simulink model "RIN251230_16_SV_H4_l2_2"  (R2018b)
settings: Solver=VariableStepAuto  StartTime=0.0  StopTime=0.2  RelTol=1e-3
libraries: powerlib x83, powerlib_meascontrol x4
settings Model: Creator=ADMINISTRATOR  LastModifiedBy=VID Company
settings SFSimCC: SimUseLocalCustomCode=off
settings RTWCC: RTWUseLocalCustomCode=off
settings CodeAppCC: StateflowObjectComments=on
settings SimscapeCC: SimscapeNormalizeSystem=off

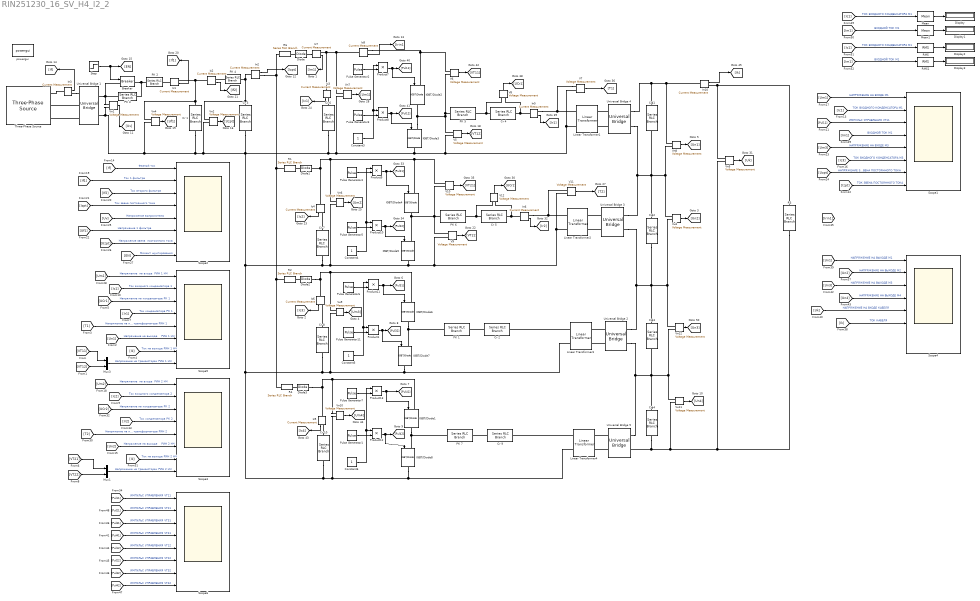
== system RIN251230_16_SV_H4_l2_2 ==
   R{1..2,4,6} (4 alike) : powerlib/Elements/Series RLC Branch  LConnTagsString=__new0  RConnTagsString=__new0  BranchType=R  Resistance=0.001  Inductance=1e-3  SetiL0=off  InitialCurrent=0  Capacitance=1e-6  Setx0=off  InitialVoltage=0  Measurements=None
      settings: SourceProductName=Simscape Electrical
  " R3" : powerlib/Elements/Series RLC Branch  LConnTagsString=__new0  RConnTagsString=__new0  BranchType=R  Resistance=100  Inductance=1e-3  SetiL0=off  InitialCurrent=0  Capacitance=1e-6  Setx0=off  InitialVoltage=0  Measurements=None
      settings: SourceProductName=Simscape Electrical
  Breaker : powerlib/Elements/Breaker  InitialState=0  SwitchingTimes="[1/60  5/60]"  External=on  BreakerResistance=0.0001  SnubberResistance=1e6  SnubberCapacitance=inf  Measurements=None  MoreParameters=on  NoBreakLoop=off
      settings: SourceProductName=Simscape Electrical
  Constant{3..6} (4 alike) : Constant
  Cr 1 : powerlib/Elements/Series RLC Branch  LConnTagsString=__new0  RConnTagsString=__new0  BranchType=C  Resistance=0.001  Inductance=5e-6  SetiL0=off  InitialCurrent=0  Capacitance=4100e-6  Setx0=off  InitialVoltage=0  Measurements=Branch voltage and current
      settings: SourceProductName=Simscape Electrical
  Cr {6..8,10} (4 alike) : powerlib/Elements/Series RLC Branch  LConnTagsString=__new0  RConnTagsString=__new0  BranchType=C  Resistance=0.001  Inductance=5e-6  SetiL0=off  InitialCurrent=0  Capacitance=120e-6  Setx0=off  InitialVoltage=0  Measurements=Branch voltage and current
      settings: SourceProductName=Simscape Electrical
  Cr {2,4..5,9} (4 alike) : powerlib/Elements/Series RLC Branch  LConnTagsString=__new0  RConnTagsString=__new0  BranchType=C  Resistance=0.001  Inductance=5e-6  SetiL0=off  InitialCurrent=0  Capacitance=1.6e-6  Setx0=off  InitialVoltage=0  Measurements=Branch voltage and current
      settings: SourceProductName=Simscape Electrical
  Cr 3 : powerlib/Elements/Series RLC Branch  LConnTagsString=__new0  RConnTagsString=__new0  BranchType=C  Resistance=0.001  Inductance=5e-6  SetiL0=off  InitialCurrent=0  Capacitance=10e-6  Setx0=off  InitialVoltage=0  Measurements=Branch voltage and current
      settings: SourceProductName=Simscape Electrical
  Diode{,1..3} (4 alike) : powerlib/Power Electronics/Diode  Ron=0.001  Lon=0  Vf=0.8  IC=0  UseSnubber=0  Rs=inf  Cs=250e-9  Measurements=off
  Display{,1..3} (4 alike) : Display
  IGBT/Diode{1..8} (8 alike) : powerlib/Power Electronics/IGBT//Diode  Ron=4.5e-6  Rs=1e5  Cs=inf  Measurements=off
      settings: SourceProductName=Simscape Electrical
  Ic{1..8} (8 alike) : powerlib/Measurements/Current Measurement  PhasorSimulation=off  OutputType=Complex  PSBequivalent=0
      settings: SourceProductName=Simscape Electrical
  Iн{2..3,5..6,10} (5 alike) : powerlib/Measurements/Current Measurement  PhasorSimulation=off  OutputType=Complex  PSBequivalent=0
      settings: SourceProductName=Simscape Electrical
  Linear Transformer{1..4} (4 alike) : powerlib/Elements/Linear Transformer  UNITS=pu  NominalPower=[ 20e3 16e3 ]  winding1=[250 1e-4 1e-7]  winding2=[500 1e-4 1e-7]  ThreeWindings=off  winding3=[3.15e+05 0.7938 0.084225]  RmLm=[1e4 1e4]  Measurements=None  DataType=off
      settings: SourceProductName=Simscape Electrical
  Mean : powerlib_meascontrol/Measurements/Mean  Freq=16000  Vinit=0  Ts=0
  Mean1 : powerlib_meascontrol/Measurements/Mean  Freq=16000  Vinit=0  Ts=0
  Mux1 : Mux  Inputs=2
  Mux3 : Mux  Inputs=2
  Product{1,7..13} (8 alike) : Product
  Pulse Generator1 : DiscretePulseGenerator  PulseType=Time based  Amplitude=20  Period=1/16e3  PulseWidth=27  PhaseDelay=1/64e3
  Pulse Generator11 : DiscretePulseGenerator  PulseType=Time based  Amplitude=20  Period=1/16e3  PulseWidth=27  PhaseDelay=3/64e3
  Pulse Generator2 : DiscretePulseGenerator  PulseType=Time based  Amplitude=20  Period=1/16e3  PulseWidth=27
  Pulse Generator3 : DiscretePulseGenerator  PulseType=Time based  Amplitude=20  Period=1/16e3  PulseWidth=27  PhaseDelay=1/32e3
  Pulse Generator4 : DiscretePulseGenerator  PulseType=Time based  Amplitude=20  Period=1/16e3  PulseWidth=27  PhaseDelay=1/32e3
  Pulse Generator5 : DiscretePulseGenerator  PulseType=Time based  Amplitude=20  Period=1/16e3  PulseWidth=27
  Pulse Generator6 : DiscretePulseGenerator  PulseType=Time based  Amplitude=20  Period=1/16e3  PulseWidth=27  PhaseDelay=1/64e3
  Pulse Generator7 : DiscretePulseGenerator  PulseType=Time based  Amplitude=20  Period=1/16e3  PulseWidth=27  PhaseDelay=3/64e3
  RMS : powerlib_meascontrol/Measurements/RMS  TrueRMS=on  Freq=16000  RMSInit=0  Ts=0
  RMS1 : powerlib_meascontrol/Measurements/RMS  TrueRMS=on  Freq=16000  RMSInit=0  Ts=0
  Scope{1..6} (6 alike) : Scope  NumInputPorts=8
  Step : Step  Time=0.03  SampleTime=0
  Three-Phase Source : powerlib/Electrical Sources/Three-Phase Source  InternalConnection=Yg  VoltagePhases=off  Voltage=380  PhaseAngle=0  Voltage_phases=[25e3 25e3 25e3]/sqrt(3)  PhaseAngles_phases=[0 -120 +120]  Frequency=50  NonIdealSource=on  SpecifyImpedance=off  Resistance=50e-3  Inductance=0.4e-3  ShortCircuitLevel=100e6  BaseVoltage=380  XRratio=7  BusType=swing  Pref=10e3  Qref=0  Prefabc=[10e3, 10e3, 10e3]  Qrefabc=[0, 0, 0]  Qmin=-inf  Qmax=inf
      settings: SourceProductName=Simscape Electrical
  Universal Bridge 1 : powerlib/Power Electronics/Universal Bridge  Arms=3  SnubberResistance=1000000  SnubberCapacitance=1e-12  Device=Diodes  Ron=1e-6  Lon=0  ForwardVoltages="[  0  0  ]"  ForwardVoltage=0  GTOparameters=[ 10e-6 , 20e-6 ]  IGBTparameters=[ 1e-6 , 2e-6 ]  Measurements=Device voltages  Measurements_2=None  converterType=Rectifier
      settings: SourceProductName=Simscape Electrical
  Universal Bridge {2..5} (4 alike) : powerlib/Power Electronics/Universal Bridge  Arms=2  SnubberResistance=1000000  SnubberCapacitance=1e-12  Device=Diodes  Ron=1e-6  Lon=0  ForwardVoltages="[  0  0  ]"  ForwardVoltage=0  GTOparameters=[ 10e-6 , 20e-6 ]  IGBTparameters=[ 1e-6 , 2e-6 ]  Measurements=None  Measurements_2=None  converterType=Rectifier
      settings: SourceProductName=Simscape Electrical
  V{5..12} (8 alike) : powerlib/Measurements/Voltage Measurement  PhasorSimulation=off  OutputType=Complex  PSBequivalent=0
      settings: SourceProductName=Simscape Electrical
  Vн{1..12} (12 alike) : powerlib/Measurements/Voltage Measurement  PhasorSimulation=off  OutputType=Complex  PSBequivalent=0
      settings: SourceProductName=Simscape Electrical
  powergui : powerlib/powergui  Priority=1  SimulationMode=Discrete  SampleTime=1e-7  frequency=60  Iterations=50  frequencyindice=0  Pbase=100e6  ErrMax=1e-4  UnitsV=kV  UnitsW=MW  buscounter=0  FunctionMessages=off  echomessages=off  EnableUseOfTLC=off  CurrentSourceSwitches=off  DisableSnubberDevices=off  DisableRonSwitches=off  DisableVfSwitches=off  DisplayEquations=off  SolverType=Tustin/Backward Euler (TBE)  Interpol=off  ExternalGateDelay=off  methode=off  Ts=100  x0status=blocks  SPID=off  SwTol=0  HookPort=off  RestoreLinks=warning  ResistiveCurrentMeasurement=off  Frange=[0:2:500]  Ylog=off  Xlog=on  ShowGrid=off  save=off  variable=ZData  structure=0  ZoomFFT=off  StartTime=0.0  cycles=1  DisplayStyle=1  fundamental=60  FreqAxis=off  MaxFrequency=1000  frequencyindicesteady=1  RmsSteady=1  display=off
  РК {1,5..7} (4 alike) : powerlib/Elements/Series RLC Branch  LConnTagsString=__new0  RConnTagsString=__new0  BranchType=RL  Resistance=0.000001  Inductance=13.6e-6  SetiL0=off  InitialCurrent=0  Capacitance=3e-6  Setx0=off  InitialVoltage=0  Measurements=None
      settings: SourceProductName=Simscape Electrical
  РК 2 : powerlib/Elements/Series RLC Branch  LConnTagsString=__new0  RConnTagsString=__new0  BranchType=RL  Resistance=1e-3  Inductance=1e-3  SetiL0=off  InitialCurrent=0  Capacitance=3e-6  Setx0=off  InitialVoltage=0  Measurements=None
      settings: SourceProductName=Simscape Electrical
  РК 3 : powerlib/Elements/Series RLC Branch  LConnTagsString=__new0  RConnTagsString=__new0  BranchType=RL  Resistance=2  Inductance=1e-6  SetiL0=off  InitialCurrent=0  Capacitance=3e-6  Setx0=off  InitialVoltage=0  Measurements=None
      settings: SourceProductName=Simscape Electrical
  РК 4 : powerlib/Elements/Series RLC Branch  LConnTagsString=__new0  RConnTagsString=__new0  BranchType=RL  Resistance=1e-3  Inductance=10e-6  SetiL0=off  InitialCurrent=0  Capacitance=3e-6  Setx0=off  InitialVoltage=0  Measurements=None
      settings: SourceProductName=Simscape Electrical
  Сф{1..4} (4 alike) : powerlib/Elements/Series RLC Branch  LConnTagsString=__new0  RConnTagsString=__new0  BranchType=C  Resistance=0.001  Inductance=5e-6  SetiL0=off  InitialCurrent=0  Capacitance=60e-6  Setx0=off  InitialVoltage=300  Measurements=Branch voltage and current
      settings: SourceProductName=Simscape Electrical
  wires:
  [UCr1] -> Scope5/3  "Напряжение на конденсаторе РК 1"
  [Ik] -> Scope5/7  "Ток на выходе РИН 1 НЧ"
  [Un1] -> Scope5/6  "Напряжение на выходе    РИН 1 НЧ"
  [T1] -> Scope5/5  "Напряжение на первичной обмотке трансформатора РИН 1"
  [Ir1] -> Scope5/4  "Ток конденсатора РК 1"
  Iн2/1 -> [Izpt]
  [Ic1] -> Scope5/2  "Ток входного конденсатора 1"
  Iн3/1 -> [If]
  Step/1 -> [EN], Breaker/1
  Vн2/1 -> [Uzpt]
  Vн4/1 -> [Uf1]
  Vн1/1 -> [Uv]
  Ic1/1 -> [If1]
  Ic2/1 -> [If2]
  [If] -> Scope2/1  "Фазный ток"
  [If1] -> Scope2/2  "Ток 1 фильтра"
  [If2] -> Scope2/3  "Ток второго фильтра"
  [Izpt] -> Scope2/4  "Ток звена постоянного тока"
  [Uv] -> Scope2/5  "Напряжение выпрямителя"
  [Uf1] -> Scope2/6  "Напряжение 1 фильтра"
  [Uzpt] -> Scope2/7  "Напряжение звена  постоянного тока"
  [EN] -> Scope2/8  "Момент шунтирования"
  [Um1] -> Scope5/1  "Напряжение  на входе  РИН 1 НЧ"
  [VT12] -> Mux3/2
  [VT11] -> Mux3/1
  Mux3/1 -> Scope5/8  "Напряжение на транзисторах РИН 1 НЧ"
  V6/1 -> [VT11]
  V5/1 -> [VT12]
  Vн5/1 -> [Uk]
  V7/1 -> [T1]
  V8/1 -> [UCr1]
  Iн5/1 -> [Ir1]
  Product8/1 -> IGBT/Diode3/1, [Pul12]
  Product7/1 -> IGBT/Diode2/1, [Pul11]
  Ic3/1 -> [Ic1]
  Pulse Generator2/1 -> Product7/2
  Pulse Generator3/1 -> Product8/2
  Constant3/1 -> Product7/1, Product8/1
  Vн7/1 -> [Um1]
  V10/1 -> [VT21]
  V9/1 -> [VT22]
  V11/1 -> [T2]
  V12/1 -> [UCr2]
  Iн6/1 -> [Ir2]
  Product10/1 -> IGBT/Diode5/1, [Pul22]
  Product9/1 -> IGBT/Diode4/1, [Pul21]
  Ic4/1 -> [Ic2]
  Pulse Generator4/1 -> Product9/2
  Pulse Generator5/1 -> Product10/2
  Constant4/1 -> Product9/1, Product10/1
  Vн6/1 -> [Um2]
  Vн8/1 -> [Un1]
  Vн3/1 -> [Un2]
  Iн10/1 -> [Ik]
  [UCr2] -> Scope3/3  "Напряжение на конденсаторе РК 2"
  [Ik] -> Scope3/7  "Ток на выходе РИН 2 НЧ"
  [Un2] -> Scope3/6  "Напряжение на выходе    РИН 2 НЧ"
  [T2] -> Scope3/5  "Напряжение на первичной обмотке трансформатора РИН 2"
  [Ir2] -> Scope3/4  "Ток конденсатора РК 2"
  [Ic2] -> Scope3/2  "Ток входного конденсатора 2"
  [Um2] -> Scope3/1  "Напряжение  на входе  РИН 2 НЧ"
  [VT22] -> Mux1/2
  [VT21] -> Mux1/1
  Mux1/1 -> Scope3/8  "Напряжение на транзисторах РИН 2 НЧ"
  Product1/1 -> [Pul32], IGBT/Diode7/1
  Product11/1 -> IGBT/Diode6/1, [Pul31]
  Ic6/1 -> [Ic3]
  Pulse Generator6/1 -> Product11/2
  Pulse Generator11/1 -> Product1/2
  Constant5/1 -> Product11/1, Product1/1
  Vн9/1 -> [Um3]
  Product12/1 -> [Pul42], IGBT/Diode8/1
  Product13/1 -> [Pul41], IGBT/Diode1/1
  Ic5/1 -> [Ic4]
  Pulse Generator7/1 -> Product13/2
  Pulse Generator1/1 -> Product12/2
  Constant6/1 -> Product13/1, Product12/1
  Vн10/1 -> [Um4]
  Vн12/1 -> [Un3]
  Vн11/1 -> [Un4]
  [Pul11] -> Scope1/3  "ИМПУЛЬС УПРАВЛЕНИЯ VT11"
  [Uzpt] -> Scope1/7  "НАПРЯЖЕНИЕ ЗВЕНА ПОСТОЯННОГО ТОКА"
  [Ic3] -> Scope1/6  "ТОК ВХОДНОГО КОНДЕНСАТОРА М3"
  [Um3] -> Scope1/5  "НАПРЯЖЕНИЕ НА ВХОДЕ М3"
  [Im1] -> Scope1/4  "ВХОДНОЙ ТОК М1"
  [Ic1] -> Scope1/2  "ТОК ВХОДНОГО КОНДЕНСАТОРА М1"
  [Um1] -> Scope1/1  "НАПРЯЖЕНИЕ НА ВХОДЕ М1"
  [Un3] -> Scope4/3  "НАПРЯЖЕНИЕ НА ВЫХОДЕ М3"
  [Ik] -> Scope4/6  "ТОК КАБЕЛЯ"
  [Uk] -> Scope4/5  "НАПРЯЖЕНИЕ НА ВХОДЕ КАБЕЛЯ"
  [Un4] -> Scope4/4  "НАПРЯЖЕНИЕ НА ВЫХОДЕ М4"
  [Un2] -> Scope4/2  "НАПРЯЖЕНИЕ НА ВЫХОДЕ М2"
  [Un1] -> Scope4/1  "НАПРЯЖЕНИЕ НА ВЫХОДЕ М1"
  [Izpt] -> Scope1/8  "ТОК ЗВЕНА ПОСТОЯННОГО ТОКА"
  Ic7/1 -> [Im1]
  [Pul11] -> Scope6/1  "ИМПУЛЬС УПРАВЛЕНИЯ VT11"
  [Pul21] -> Scope6/2  "ИМПУЛЬС УПРАВЛЕНИЯ VT21"
  [Pul41] -> Scope6/4  "ИМПУЛЬС УПРАВЛЕНИЯ VT41"
  [Pul31] -> Scope6/3  "ИМПУЛЬС УПРАВЛЕНИЯ VT31"
  [Pul12] -> Scope6/5  "ИМПУЛЬС УПРАВЛЕНИЯ VT12"
  [Pul22] -> Scope6/6  "ИМПУЛЬС УПРАВЛЕНИЯ VT22"
  [Pul32] -> Scope6/7  "ИМПУЛЬС УПРАВЛЕНИЯ VT32"
  [Pul42] -> Scope6/8  "ИМПУЛЬС УПРАВЛЕНИЯ VT42"
  Ic8/1 -> [Irin1]
  [Ic1] -> Mean/1  "ТОК ВХОДНОГО КОНДЕНСАТОРА М1"
  [Im1] -> Mean1/1  "ВХОДНОЙ ТОК М1"
  Mean/1 -> Display/1
  Mean1/1 -> Display1/1
  RMS/1 -> Display2/1
  RMS1/1 -> Display3/1
  [Ic1] -> RMS/1  "ТОК ВХОДНОГО КОНДЕНСАТОРА М1"
  [Im1] -> RMS1/1  "ВХОДНОЙ ТОК М1"
  connections:
  РК 2/LConn1 -- Breaker/RConn1 -- РК 3/RConn1
  Universal Bridge 1/LConn3 -- Three-Phase Source/RConn3
  Universal Bridge 1/LConn2 -- Three-Phase Source/RConn2
  Iн3/LConn1 -- Three-Phase Source/RConn1
  Iн3/RConn1 -- Universal Bridge 1/LConn1
  Universal Bridge 1/RConn1 -- Vн1/LConn1 -- РК 3/LConn1 -- Breaker/LConn1
  Cr 1/LConn1 -- Vн4/LConn1 -- Ic2/LConn1 -- Ic1/RConn1
  Ic1/LConn1 -- РК 2/RConn1
  РК 4/LConn1 -- Ic2/RConn1
  IGBT/Diode3/LConn1 -- V6/LConn2 -- РК 5/LConn1 -- V5/LConn1 -- IGBT/Diode2/RConn1
  Iн5/LConn1 -- Cr 4/RConn1 -- V8/LConn2
  РК 5/RConn1 -- V8/LConn1 -- Cr 4/LConn1
  V7/LConn1 -- Iн5/RConn1 -- Linear Transformer1/LConn1
  IGBT/Diode3/RConn1 -- Linear Transformer1/LConn2 -- V7/LConn2 -- V5/LConn2 -- Linear Transformer3/LConn2 -- IGBT/Diode7/RConn1 -- Vн9/LConn2 -- Cr 8/RConn1 -- Cr 10/RConn1 -- Linear Transformer4/LConn2 -- IGBT/Diode8/RConn1 -- Vн10/LConn2 -- V11/LConn2 -- Linear Transformer2/LConn2 -- V9/LConn2 -- IGBT/Diode5/RConn1 -- Vн6/LConn2 -- Cr 7/RConn1 -- Cr 1/RConn1 -- Vн1/LConn2 -- Universal Bridge 1/RConn2 -- Vн4/LConn2 -- Vн2/LConn2 -- Cr 3/RConn1 -- Cr 6/RConn1 -- Vн7/LConn2
  V6/LConn1 -- IGBT/Diode2/LConn1 -- Ic8/RConn1
  V12/LConn2 -- Iн6/LConn1 -- Cr 5/RConn1
  Cr 5/LConn1 -- РК 6/RConn1 -- V12/LConn1
  Linear Transformer2/LConn1 -- V11/LConn1 -- Iн6/RConn1
  Сф2/RConn1 -- Сф3/LConn1 -- Universal Bridge 2/RConn1 -- Universal Bridge 3/RConn2 -- Vн12/LConn1 -- Vн3/LConn2
  Ic4/LConn1 -- Diode1/RConn1 -- Vн6/LConn1 -- V10/LConn1 -- IGBT/Diode4/LConn1
  Universal Bridge 3/RConn1 -- Universal Bridge 4/RConn2 -- Vн3/LConn1 -- Vн8/LConn2 -- Сф2/LConn1 -- Сф1/RConn1
  Universal Bridge 4/LConn2 -- Linear Transformer1/RConn2
  Cr 7/LConn1 -- Ic4/RConn1
  Universal Bridge 4/LConn1 -- Linear Transformer1/RConn1
  Cr 6/LConn1 -- Ic3/RConn1
  Universal Bridge 3/LConn1 -- Linear Transformer2/RConn1
  Universal Bridge 3/LConn2 -- Linear Transformer2/RConn2
  IGBT/Diode4/RConn1 -- IGBT/Diode5/LConn1 -- V9/LConn1 -- РК 6/LConn1 -- V10/LConn2
  Universal Bridge 4/RConn1 -- Iн10/LConn1 -- Vн8/LConn1 -- Сф1/LConn1
  Vн5/LConn1 -- " R3"/LConn1 -- Iн10/RConn1
  Cr 2/LConn1 -- РК 1/RConn1
  Vн9/LConn1 -- Diode2/RConn1 -- Ic6/LConn1 -- IGBT/Diode6/LConn1
  IGBT/Diode6/RConn1 -- IGBT/Diode7/LConn1 -- РК 1/LConn1
  Cr 8/LConn1 -- Ic6/RConn1
  Universal Bridge 2/LConn1 -- Linear Transformer3/RConn1
  Universal Bridge 2/LConn2 -- Linear Transformer3/RConn2
  Cr 9/LConn1 -- РК 7/RConn1
  Ic5/LConn1 -- Diode3/RConn1 -- Vн10/LConn1 -- IGBT/Diode1/LConn1
  РК 7/LConn1 -- IGBT/Diode8/LConn1 -- IGBT/Diode1/RConn1
  Universal Bridge 5/LConn1 -- Linear Transformer4/RConn1
  Universal Bridge 5/LConn2 -- Linear Transformer4/RConn2
  Cr 10/LConn1 -- Ic5/RConn1
  Сф4/LConn1 -- Сф3/RConn1 -- Vн12/LConn2 -- Vн11/LConn1 -- Universal Bridge 2/RConn2 -- Universal Bridge 5/RConn1
  " R3"/RConn1 -- Vн11/LConn2 -- Сф4/RConn1 -- Universal Bridge 5/RConn2 -- Vн5/LConn2
  Linear Transformer4/LConn1 -- Cr 9/RConn1
  Linear Transformer3/LConn1 -- Cr 2/RConn1
  Iн2/RConn1 -- " R4"/LConn1 -- " R2"/LConn1 -- " R1"/LConn1 -- " R6"/LConn1
  РК 4/RConn1 -- Cr 3/LConn1 -- Vн2/LConn1 -- Iн2/LConn1
  Ic7/RConn1 -- Ic8/LConn1 -- Vн7/LConn1 -- Ic3/LConn1
  Diode/LConn1 -- " R6"/RConn1
  Diode/RConn1 -- Ic7/LConn1
  Diode1/LConn1 -- " R1"/RConn1
  Diode2/LConn1 -- " R2"/RConn1
  Diode3/LConn1 -- " R4"/RConn1
